simulink model "Oving3Oppg3c"  (R2020b)
settings: Solver=VariableStepAuto  StartTime=0.0  StopTime=1000  MaxStep=0.01  RelTol=1e-3
values from neighbouring files (symbols this model uses):
  A = 2.34    [Oving3Oppg3Variables.mat]
  C_d = 0.24    [Oving3Oppg3Variables.mat]
  d = 0    [Oving3Oppg3Variables.mat]
  m = 2170    [Oving3Oppg3Variables.mat]
  rho = 1.225    [Oving3Oppg3Variables.mat]
  v_0 = 25    [Oving3Oppg3Variables.mat]
settings Model: Creator=crezl  LastModifiedBy=crezl

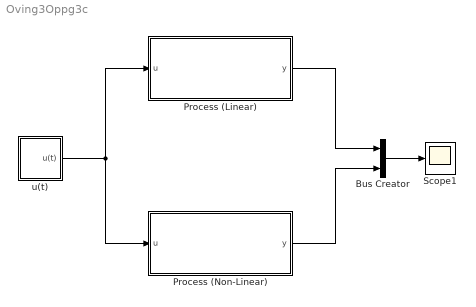
== system Oving3Oppg3c ==
  Bus Creator : BusCreator  Inputs=2
  Process (Linear) : Subsystem
  Process (Non-Linear) : Subsystem
  Scope1 : Scope
  u(t) : Subsystem
  wires:
  Process (Linear)/1(y) -> Bus Creator/1
  u(t)/1(u(t)) -> Process (Linear)/1(u), Process (Non-Linear)/1(u)
  Bus Creator/1 -> Scope1/1
  Process (Non-Linear)/1(y) -> Bus Creator/2

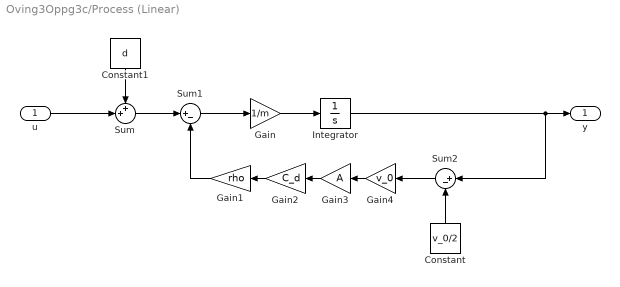
== system Oving3Oppg3c/Process (Linear) ==
  u : Inport
  Constant : Constant  Value=v_0/2
  Constant1 : Constant  Value=d
  Gain : Gain  Gain=1/m
  Gain1 : Gain  Gain=rho
  Gain2 : Gain  Gain=C_d
  Gain3 : Gain  Gain=A
  Gain4 : Gain  Gain=v_0
  Integrator : Integrator  InitialCondition=v_0*1.2
  Sum : Sum  Inputs=++|
  Sum1 : Sum  Inputs=|+-
  Sum2 : Sum  Inputs=|+-
  y : Outport
  wires:
  Constant1/1 -> Sum/1
  Integrator/1 -> Sum2/1, y/1
  Sum/1 -> Sum1/1
  Gain1/1 -> Sum1/2
  Sum1/1 -> Gain/1
  Gain3/1 -> Gain2/1
  Gain2/1 -> Gain1/1
  Gain/1 -> Integrator/1
  u/1 -> Sum/2
  Gain4/1 -> Gain3/1
  Constant/1 -> Sum2/2
  Sum2/1 -> Gain4/1

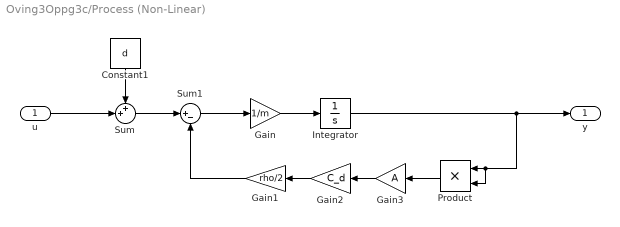
== system Oving3Oppg3c/Process (Non-Linear) ==
  u : Inport
  Constant1 : Constant  Value=d
  Gain : Gain  Gain=1/m
  Gain1 : Gain  Gain=rho/2
  Gain2 : Gain  Gain=C_d
  Gain3 : Gain  Gain=A
  Integrator : Integrator  InitialCondition=v_0*1.2
  Product : Product
  Sum : Sum  Inputs=++|
  Sum1 : Sum  Inputs=|+-
  y : Outport
  wires:
  Constant1/1 -> Sum/1
  Integrator/1 -> y/1, Product/2, Product/1
  Sum/1 -> Sum1/1
  Gain1/1 -> Sum1/2
  Sum1/1 -> Gain/1
  Product/1 -> Gain3/1
  Gain3/1 -> Gain2/1
  Gain2/1 -> Gain1/1
  Gain/1 -> Integrator/1
  u/1 -> Sum/2

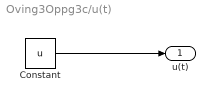
== system Oving3Oppg3c/u(t) ==
  Constant : Constant  Value=u
  u(t) : Outport
  wires:
  Constant/1 -> u(t)/1
